simulink model "Prediction_3sAdvance_2output"  (R2016b)
settings: Solver=FixedStepAuto  StartTime=0.0  StopTime=length(lat_y)  FixedStep=1  RelTol=1e-3
StopFcn:
  | %%
  | scrsz = get(groot,'ScreenSize');
  | figure('Position',[40 scrsz(4)*0.1 scrsz(3)*0.8 scrsz(4)*0.8])
  | 
  | lng_margin = (max(LOCATIONLongitude(indices))-min(LOCATIONLongitude(indices)))*0.01;
  | lat_margin = (max(LOCATIONLatitude(indices))-min(LOCATIONLatitude(indices)))*0.01;
  | 
  | live_plot_title = ['Pedestrian Path Neural Network Prediction' newline ...
  |     'Green Rectangle:Current Position, Cyan Rectangle:Future Position' newline ...
  |     'blue line:predicted, green line:actual path'];
  | 
  | %occupy space on google map to plot the predicted trajectory
  | annotation('textbox', [0.7 0.9 0.1 0.1],'String', live_plot_title,'EdgeColor', 'k','HorizontalAlignment', 'center','FontWeight','bold');
  | 
  | %plot for acutal pedestrian path
  | subplot(1,2,1);
  | actual_lng = LOCATIONLongitude(indices);
  | actual_lat = LOCATIONLatitude(indices);
  | plot(actual_lng,actual_lat,'g','linewidth',2); hold on;
  | plot_google_map('MapType','satellite');
  | xlim([min(actual_lng)-lng_margin max(actual_lng)+lng_margin]);
  | ylim([min(actual_lat)-lat_margin max(actual_lat)+lat_margin]);
  | title('Actual Pedestrian Path');xlabel('Longitude');ylabel('Latitude');
  | 
  | 
  | predict_y = out_x.signals.values;
  | predict_x = out_y.signals.values;
  | 
  | %convert the predicted path to the latitude and longitude
  | [predict_lat,predict_lng] = utm2ll(predict_y + x_init, predict_x + y_init,zone);
  | subplot(1,2,2);
  | title('Predicted Pedestrian Path');xlabel('Longitude');ylabel('Latitude');
  | lat_lim = [min(predict_lat) min(predict_lat) max(predict_lat) max(predict_lat)];
  | long_lim = [max(predict_lng) min(predict_lng) min(predict_lng) max(predict_lng)];
  | scatter(long_lim, lat_lim);
  | plot_google_map('MapType','satellite');
  | xlim([min(predict_lng)-lng_margin max(predict_lng)+lng_margin]);
  | ylim([min(predict_lat)-lat_margin max(predict_lat)+lat_margin]);
  | for(i=1:1:length(actual_lat))
  |     plot(actual_lng(i),actual_lat(i),'gs','MarkerSize',10);hold on;
  |     plot(predict_lng(i),predict_lat(i),'bs','MarkerSize',10);hold on;
  | 
  |     RectPosCurr = [actual_lng(i)-lng_margin*2 actual_lat(i)-lat_margin*2 lng_margin*4 lat_margin*4];
  |     RectPosFuture = [predict_lng(i)-lng_margin*2 predict_lat(i)-lat_margin*2 lng_margin*4 lat_margin*4];
  |     showCurr = rectangle('Position',RectPosCurr,'FaceColor','g','Visible','on');
  |     showFuture = rectangle('Position',RectPosFuture,'FaceColor','c','Visible','on');
  |     pause(0.01/2);
  | 
  |     set(showCurr,'Visible','off');
  |     set(showFuture,'Visible','off');
  |     pause(0.01/2);
  | end
  | 
  | 
  | save('TestData_NNPred_3s.mat','indices','LOCATIONLatitude','LOCATIONLongitude','predict_lat','predict_lng');
values from neighbouring files (symbols this model uses):
  indices = [20 21 22 23 24 25 26 27 28 29 30 31 ... (1110 elements, 1110x1)]    [Circle.mat]    (also in DoubleEllipse.mat = [57 58 59 60 61 62 63 64 65 66 67 68 ... (2382 elements, 238; GPS_Path_Prediction.m = find(~isempty(orientation_temp)&~isnan(orientation_temp)); Rectangle.mat = [51 52 53 54 55 56 57 58 59 60 61 62 ... (1700 elements, 170; special_filter.m = find(variance<=var_threshold & abs(magnitude) <= mag_thresho)
  LOCATIONLatitude = [42.32249 42.32249 42.32249 42.32249 42.32249 42.32249 42.32249 42.32249 42.32249 42.32249 42.32249 42.32249 ... (1135 elements, 1135x1)]    [Circle.mat]    (also in DoubleEllipse.mat = [42.322384 42.322384 42.322384 42.322384 42.322384 42.322384; Rectangle.mat = [42.323025 42.323025 42.323025 42.323025 42.323025 42.323025)
  LOCATIONLongitude = [-83.479965 -83.479965 -83.479965 -83.479965 -83.479965 -83.479965 -83.479965 -83.479965 -83.479965 -83.479965 -83.479965 -83.479965 ... (1135 elements, 1135x1)]    [Circle.mat]    (also in DoubleEllipse.mat = [-83.47919 -83.47919 -83.47919 -83.47919 -83.47919 -83.47919; Rectangle.mat = [-83.47979 -83.47979 -83.47979 -83.47979 -83.47979 -83.47979)
libraries: neural x17
(part 2 of 2)

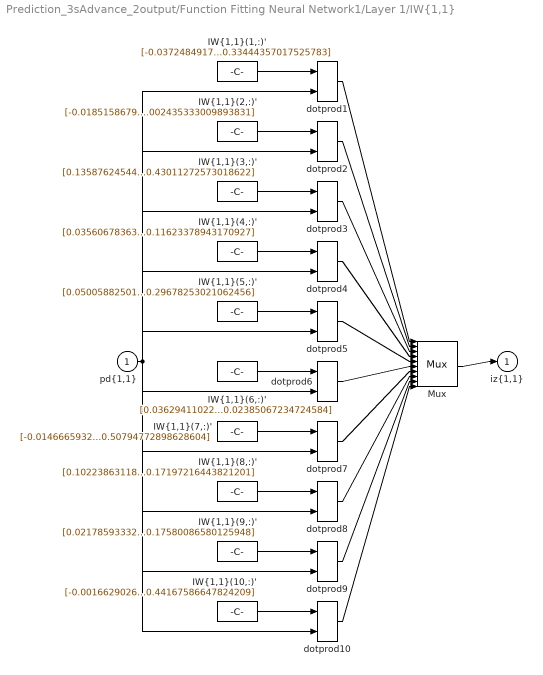
== system Prediction_3sAdvance_2output/Function Fitting Neural Network1/Layer 1/IW{1,1} ==
  "pd{1,1}" : Inport  PortDimensions=98
      mask Display: e = 0.06;c1 = [120 230 180]/255;c2 = ([120 230 180]+0)/(256+128);c3 = ([120 230 180]+128)/(256+128);patch([0 1 1 0],[0 0 1 1],c1);patch([0 1 1 1-e 1-e 0+e],[0 0 1 1-e 0+e 0+e],c2);patch([0 0 1 1-e 0+e 0+e],[0 1 1 1-e 1-e 0+e],c3);plot([0 1 1 0 0],[0 0 1 1 0]);
  "IW{1,1}(1,:)'" : Constant  Value=[-0.037248491787892045;0.0054460879972825669;-0.032907236588145455;0.0081200830673537269;0.045384948749954322;0.014503686240496656;0.03213178028993087;0.0044720544327022304;0.1328606211490925;-0.0022121594803582462;0.028994122142392876;-0.035971140027549996;0.012867042667458866;0.011984749837422535;-0.021689470658739135;-0.098691166617321593;0.013835297396100571;0.045570042540193985;0.006732817710215876;0.056374567113716509;0.043103145013547291;0.0094980051068001906;0.011375051456096234;0.044909003539689206;0.013443186350408389;0.064030515050383083;0.023608898902052266;-0.0018830103419206399;0.061923384001760527;0.099859366394465326;-0.035351467689058703;0.059571473168069197;0.050539807340897455;-0.0097345743458838955;-0.03019968727482451;-0.043083228725856432;-0.075672940267287103;-0.021341628750718045;-0.0075860255498702654;0.083882467573331537;0.087081548182975047;0.044326747243472769;0.04161843098207673;0.024419517359105761;0.067771261194288154;0.10793722049789942;0.098853911319223733;0.14510369382563093;0.14667611627198809;0.098747855953836922;0.055482620021514113;0.041358834886326398;-0.06234927403230036;0.02054383239817216;-0.0060832941492655933;-0.063800851461126837;0.025933913655796729;0.050253244099810558;0.17323753390638694;0.013583006031321749;0.047212997932893068;0.075090512042532781;0.020234443163722624;0.0096757232713807779;0.052770574120711317;0.070525108516196325;-0.038937279988646559;-0.041985340387868511;0.014003118123182268;-0.027139949440495883;0.035464437514537303;-0.020146467949284624;-0.029730945962615059;-0.033925780053117936;-0.062662865795619846;-0.073264534007386958;-0.092259914356993614;-0.12216892759248806;-0.036836270598460542;0.030334850772608789;-0.024565227656025427;-0.042277399900198631;-0.0024047230683458681;0.014120658740865528;-0.0072595459538706102;-0.061761095504444627;-0.06187148564013973;-0.10356580099254845;-0.067169875864027187;0.0070040934394714031;0.0071287719899211259;0.048236708391222453;0.037985710007260746;0.10302214241440466;0.11905881344586938;0.12569251526883041;0.16580876913423129;0.33444357017525783]
      mask Display: e = 0.06;c1 = [120 150 230]/255;c2 = ([120 150 230]+0)/383;c3 = ([120 150 230]+128)/383;patch([0 1 1 0],[0 0 1 1],c1);patch([0 1 1 1-e 1-e 0+e],[0 0 1 1-e 0+e 0+e],c2);patch([0 0 1 1-e 0+e 0+e],[0 1 1 1-e 1-e 0+e],c3);plot([0 1 1 0 0],[0 0 1 1 0]);disp('Weights');
  "IW{1,1}(10,:)'" : Constant  Value=[-0.0016629026063656727;-0.011225670780938314;0.01714849238849744;-0.014851048604781899;-0.020637093578709385;-0.0046831860505636659;0.043094815427376622;0.028144643783737999;-0.022275518567648131;-0.0054518287728863388;0.03074009069753697;0.025138591166365739;-0.0079854805933421528;-0.04352290978946536;0.0010432346396246478;0.074436831257383332;0.013522159226849562;-0.0341297472249463;0.023406280563916047;0.091245390177894556;0.03827735819353352;0.080714730073544433;0.040277637795607273;0.085186992106267831;0.0186755045141659;-0.0054963517695382066;0.0070899993972764665;0.02949082721780126;0.10821947711953832;0.10817926734261073;0.082409291320067232;0.031690910848052152;0.034667610327898127;0.0433582120696945;0.018192554323846189;0.056573488388800171;0.014924264980190824;0.020118047375342042;0.030480492656397247;-0.0058851918351701003;-0.076794887795094094;-0.055692543731693168;-0.0017313919310336671;-0.014917045039794821;0.012524053849874702;-0.078419463356555252;-0.059764956528005418;-0.028141054435656503;0.018383017379927775;0.025443583353570727;0.010694989338841221;0.0039818411387992731;0.042809605088047722;0.018337051314347801;-0.046626196567637515;0.0037444246905761658;-0.0020405572060482255;-0.043748333162415151;-0.060780149752281694;-0.0039068518534030299;0.05896696454326298;-0.02863175170986388;0.033266447694883572;0.041622866817240853;-0.08954756202660849;0.017972498221519192;0.03390177197352804;0.054709382453847911;0.05433729818294214;-0.0042915113923628718;-0.047063935588578409;-0.02706499899996518;-0.057794788791328849;-0.015379845884019749;0.022895306638709489;0.057993731050136714;0.078958851033474553;0.054172104572487355;0.038357924322599282;-0.083992107272182537;-0.072266815919457758;6.1798772163990078e-06;-0.07081353241630664;0.010229098049463453;0.018436384686728997;0.073894448949775676;0.029146559047782367;0.053097005701577576;0.02592954461261476;-0.1392726539051789;-0.078387592068944786;-0.09554649128959955;-0.12874955344751221;-0.10226641047758218;-0.15107489556282452;-0.16648423347524063;-0.2708673890968582;-0.44167586647824209]
      mask Display: e = 0.06;c1 = [120 150 230]/255;c2 = ([120 150 230]+0)/383;c3 = ([120 150 230]+128)/383;patch([0 1 1 0],[0 0 1 1],c1);patch([0 1 1 1-e 1-e 0+e],[0 0 1 1-e 0+e 0+e],c2);patch([0 0 1 1-e 0+e 0+e],[0 1 1 1-e 1-e 0+e],c3);plot([0 1 1 0 0],[0 0 1 1 0]);disp('Weights');
  "IW{1,1}(2,:)'" : Constant  Value=[-0.018515867974339798;0.0076899503655227701;0.01549069700479022;-0.0056572792377067574;-0.012941296175993957;0.0033684867282773841;-0.058734471901459022;-0.081499585394107829;-0.028289002835481376;-0.035714857870032694;0.025667867232901032;0.04701972373377955;-0.0042133746724056231;-0.040939734469384641;-0.081541047904027775;-0.035294479381303055;-0.025241872221598939;-0.044003899699484886;-0.061673568167941999;0.014271729195278368;0.039251376410087781;0.046993966092720267;-0.063891609263935056;-0.11313163856257076;-0.1658771793661056;-0.1489984542371538;-0.16679995745427703;-0.17934041911962106;-0.18280513882114119;-0.095936524801705836;-0.10069152341246847;-0.1258890389605237;-0.13539267595915977;-0.14402495236540552;-0.14208356430789368;-0.072830778023318485;-0.076229572602964174;-0.10200974763478331;-0.117850729273751;-0.024398371894119707;-0.061402312879435587;-0.05651051475020305;-0.00051209801424940873;0.0092792497807744866;0.031976932064244019;0.039163231932612605;0.10355035046087578;0.12284960076201655;0.21158867218529864;0.047482784905967378;0.065228424745243402;0.059897782952027571;0.080226172123634795;0.05566470801791959;0.090706225979411734;0.098944867731393382;0.068905625794264777;0.13976145424980396;0.21131314081599267;0.031745391815384078;-0.05505276308827943;0.014293117061868588;0.037198339502602117;0.062758768804144868;0.054681783297909493;0.051666561584193318;0.081668971795550535;0.11462921442882772;0.32986386475644031;0.036997138688802785;-0.013181832862036565;0.084037248324108471;0.057756839501518713;0.07889037953955623;0.0601386369901451;0.1018222445144861;0.13245023014536811;0.14926602137580236;0.24387994631514523;-0.058033518135738198;-0.045295437203196974;0.010683605378673021;-0.021991667219666146;0.0040487227994625485;-0.0072522018112378267;-0.0055938145531558405;0.04381260203260922;0.084441879469903974;0.25644765403914432;0.008448357593588399;0.024022196258855592;0.028951585693181837;0.042038473618834865;0.032302074150262969;0.026838544911972895;0.045227883905683615;0.073032635761526549;0.002435333009893831]
      mask Display: e = 0.06;c1 = [120 150 230]/255;c2 = ([120 150 230]+0)/383;c3 = ([120 150 230]+128)/383;patch([0 1 1 0],[0 0 1 1],c1);patch([0 1 1 1-e 1-e 0+e],[0 0 1 1-e 0+e 0+e],c2);patch([0 0 1 1-e 0+e 0+e],[0 1 1 1-e 1-e 0+e],c3);plot([0 1 1 0 0],[0 0 1 1 0]);disp('Weights');
  "IW{1,1}(3,:)'" : Constant  Value=[0.13587624544436069;0.049141070836930784;0.055226063647529307;-0.012024336315060894;0.029034721842293155;-0.0041841553803683021;-0.065110590519533496;-0.0050635145871141983;0.040305530529815912;-0.085086041805926646;-0.090753085285472365;-0.094194634308307393;-0.039192722872914643;-0.059810066311579785;0.015513472748620655;0.012009275529506782;-0.043981807150994111;-0.077587265971912206;-0.15548998679938819;-0.24987403328526672;-0.19804084126057198;-0.17565913085640739;-0.13977601925396552;-0.071775633359446422;-0.040272835600189856;-0.11407745658720843;-0.098303028907055404;-0.17288751490833559;-0.10522065490498507;-0.089892967049061634;-0.15403131387778668;-0.081779937720551907;-0.022034426415758288;0.01884725625518004;0.052770277999356845;0.03093008030701113;0.056756580220202753;0.06594354634264267;0.11632598695950128;0.068516598550003124;0.059536393304533461;0.092129347320588584;0.074913709596080291;0.054430210300128457;0.087264558634397277;0.079091055803260479;0.085051401799193779;0.037287353311588854;0.012666539134766626;-0.14012020554181653;-0.070051334847068603;-0.060773831053804538;0.013004994380231298;-0.014008098862541172;-0.037936218923967369;0.027244013025779147;-0.081009048385727381;-0.20417535790813271;-0.27273542717959298;-0.21118048832315597;-0.15657079304813487;-0.19154348051272566;-0.072217831691342022;-0.13419605969815465;-0.14409080429035978;-0.12215260942387618;-0.14080449342729862;-0.19174355199966939;-0.23874205581689281;-0.16896536250349556;-0.040501233782424088;0.04537096254121948;0.042332264815653019;0.063687965094504848;0.077026072108855481;0.053709327467266456;0.060106009911613419;-0.064670249270740748;-0.13381377122772231;-0.05098124119250879;-0.066430488971651713;-0.049535474912235977;0.00080231968539829109;-0.0090958125907286101;0.017502750704307284;0.0020256960728958001;0.013103620510808203;0.0018794618550559456;-0.1215060955417776;0.032972428012565801;0.020483431157685944;0.11723962277897426;0.11107314470112689;0.1874335444319373;0.23392080161571363;0.28071306377543098;0.36536466962570419;0.43011272573018622]
      mask Display: e = 0.06;c1 = [120 150 230]/255;c2 = ([120 150 230]+0)/383;c3 = ([120 150 230]+128)/383;patch([0 1 1 0],[0 0 1 1],c1);patch([0 1 1 1-e 1-e 0+e],[0 0 1 1-e 0+e 0+e],c2);patch([0 0 1 1-e 0+e 0+e],[0 1 1 1-e 1-e 0+e],c3);plot([0 1 1 0 0],[0 0 1 1 0]);disp('Weights');
  "IW{1,1}(4,:)'" : Constant  Value=[0.035606783631557504;-8.7920307566643552e-05;0.0077959643954650546;-0.026902507046974191;0.055430121324307691;-0.0081937769022633663;-0.019906801603008572;-0.017565781502400554;0.046813991938548988;-0.073208601225467254;-0.10161323200571563;-0.051330837516489369;-0.029012281240574062;-0.028052294075657895;-0.018270161675946285;-0.013769543175600253;0.022778808438588219;-0.0095418727838311856;-0.062534520451273667;-0.16162860103322177;-0.02839125452697229;0.038818876936792902;-0.0034962790707465663;0.044851793895644948;0.053178207180812023;0.061990968774601696;0.0050446935402055117;0.034178699305044177;0.10588014417961089;0.11956326788531846;0.20425031405267235;0.16405606467873152;0.14610633738655016;0.089798683528575618;0.087418745285612706;0.11500260140373852;0.079470205850699929;0.078160405812048944;0.027900751607239337;-0.025560766232941436;-0.094090816072839339;-0.042141551991293769;0.05901639672500518;0.040691879475591532;0.053787363822609929;0.042216007208548054;0.048387673558473156;0.06913261163375907;0.17816067291969345;0.1576713185227645;0.129922067015072;0.091200864970768583;0.060930988606987577;-0.010956761961097973;-0.055311056542727971;-0.011132434687715144;-0.06153535590517608;-0.13243463095951369;-0.19955970730551983;-0.22576929138787585;-0.23540660909952371;-0.14674720590313747;-0.12240047820282718;-0.10030002370112973;-0.10542871583418527;-0.14521324073126471;-0.17844998778519686;-0.36677533336408641;-0.33823936016763789;-0.29129894211593388;-0.289332280800773;-0.14220850820429379;-0.074582999652055337;-0.026680447939382124;-0.025778906285101599;0.004118716095315918;0.038496711872225468;-0.027659718751088871;0.0021762711750338737;-0.075576255254093186;-0.079810477521530282;-0.027772881627048111;0.012499026698608027;0.0082000081123978861;0.021694798721866596;-0.045196876928365388;-0.057483619182821417;-0.17512680000426883;-0.098411581131589446;-0.1837414194972174;-0.16401189957762166;-0.083125834629177095;-0.037564988463133393;-0.0064697206246631736;0.038046316375805488;0.053795825287118244;0.12973921102539035;0.11623378943170927]
      mask Display: e = 0.06;c1 = [120 150 230]/255;c2 = ([120 150 230]+0)/383;c3 = ([120 150 230]+128)/383;patch([0 1 1 0],[0 0 1 1],c1);patch([0 1 1 1-e 1-e 0+e],[0 0 1 1-e 0+e 0+e],c2);patch([0 0 1 1-e 0+e 0+e],[0 1 1 1-e 1-e 0+e],c3);plot([0 1 1 0 0],[0 0 1 1 0]);disp('Weights');
  "IW{1,1}(5,:)'" : Constant  Value=[0.050058825015330911;-0.0012653357721514285;0.034538905386114961;-0.0089377606265996241;0.00055185457157450263;0.028716340601122294;0.0079801906407940843;-0.045495655449408194;0.04903212752361312;-0.047442584364412857;0.01085405496138791;0.0039696743675070832;-0.10829696423943963;-0.11507296417008533;-0.1006916187242117;0.0072304873193762137;-0.0070198038464520359;-0.058760057489889314;0.065398623164374031;-0.035917083519191803;0.090562676150389973;0.10629228243770851;0.13429765641439287;0.10386240164693279;0.080837948128385781;0.022881057251614375;-0.021947611530623124;-0.021804302133922027;0.031072942275778778;-0.030446063342793282;-0.046646560789431871;-0.051629542562774168;-0.10581820304031463;-0.10980173691570538;-0.1308964798291026;-0.11654761923600809;-0.15267299201235127;-0.19546925099837423;-0.1140607288398868;-0.16559458645982331;-0.11283372853679467;-0.15367774445276097;-0.13635651783919578;-0.13753467451910104;-0.16584243315924277;-0.20303921452976351;-0.19214584685777183;-0.20321570190551377;-0.2776534551460817;-0.076180181496674992;-0.0025473866008764207;-0.071256638356988464;-0.014511365516534787;-0.026343766353206868;-0.055592068601036562;-0.039438910382926677;0.061541863800963992;0.048610001792157485;0.091072450948841421;0.015934665249430765;0.10721414601118008;0.12562602488722199;0.14617648697997296;0.14263743933781659;0.10361942488141937;0.16493857129751177;0.10064361611254671;0.10079502539515492;0.10869762397888007;0.0047085706518816767;-0.063207516262324653;-0.046679095438830011;-0.078800897801957731;-0.01925828839950719;-0.047901379372930791;-0.0096809452421214772;-0.033614754970806057;-0.002206098422528821;-0.042678487021817341;-0.11895473493421167;-0.13687664413830325;-0.10335031570448305;-0.092631636400148681;-0.050061928334915504;-0.11271154498971278;-0.053842161967614918;-0.12242795825287427;-0.11491296239191061;-0.22589475667958445;-0.19236680779187967;-0.25336304729864562;-0.24421160985511464;-0.23141079538680667;-0.22523512984473629;-0.21502591155537285;-0.32113772116854561;-0.31342712333284961;-0.29678253021062456]
      mask Display: e = 0.06;c1 = [120 150 230]/255;c2 = ([120 150 230]+0)/383;c3 = ([120 150 230]+128)/383;patch([0 1 1 0],[0 0 1 1],c1);patch([0 1 1 1-e 1-e 0+e],[0 0 1 1-e 0+e 0+e],c2);patch([0 0 1 1-e 0+e 0+e],[0 1 1 1-e 1-e 0+e],c3);plot([0 1 1 0 0],[0 0 1 1 0]);disp('Weights');
  "IW{1,1}(6,:)'" : Constant  Value=[0.036294110222280872;0.078796170074379418;0.048579716180394333;0.029244289310192888;0.027235092150712778;-0.030910566415148638;0.017589938715635575;0.077819079739231134;-0.0087185733058806197;0.0591595756626003;0.056277493880665538;0.068157807676395232;0.050072802450685336;0.0097377108828926393;-0.031357303137711512;0.040642525817573424;-0.019248081557384038;-0.0086311121682575327;-0.020976097996898403;-4.6612556843254944e-05;-0.016810053016620433;0.0011561770047757039;0.017340944138721202;-0.078866235730541398;-0.038973312525601302;-0.0021077233607033358;0.012216620132754341;0.11624884392460327;0.042525343289492465;0.00024963568421166633;0.097958686716235296;0.1044896119302359;0.074990858249646644;0.11753114014379942;0.14255312823070079;0.081536858660906902;0.11980864283949615;0.076464811217018272;0.11768083912366178;0.053040433000220877;0.071542565445890854;0.061184181214343838;0.068580045901338774;0.099053311571738051;0.067280443208284496;0.0071160854619471033;0.071633156194151087;0.050254524522790618;-0.1014827265327712;0.0077724080884053288;0.070219712452766245;0.045465455503656306;0.056391447889002279;-0.064793048136742276;0.0012113752311697468;-0.038150134401662879;-0.01917238666721521;0.035633616365967694;0.19173575257637138;0.10452066769211536;0.12306242916831635;0.0060892433529251564;-0.06482453628030875;-0.043758854212717552;0.059853881679656544;-0.020055661521191984;-0.11209882517192202;0.048397432977859686;-0.0014509675925307632;0.20499538105893558;0.11073499106249445;0.045751816712932734;-0.0073100694836159595;0.016905267946539196;0.12547688935575135;0.081686821840325552;0.085734675567429738;0.17620328903462648;0.1419606959089677;0.31580355105961361;0.29109174981011676;0.19899188574266435;0.21220310319535698;0.18750974150709493;0.15162092687987438;0.17150096652082733;0.086742438842789121;0.10228914434293929;-0.043299135787548855;0.24154249671365025;0.04904282370421801;0.009683197058250808;-0.034369901884648654;-0.12233370651460945;-0.032940987140248568;-0.14288660333844619;-0.10571383263686063;-0.02385067234724584]
      mask Display: e = 0.06;c1 = [120 150 230]/255;c2 = ([120 150 230]+0)/383;c3 = ([120 150 230]+128)/383;patch([0 1 1 0],[0 0 1 1],c1);patch([0 1 1 1-e 1-e 0+e],[0 0 1 1-e 0+e 0+e],c2);patch([0 0 1 1-e 0+e 0+e],[0 1 1 1-e 1-e 0+e],c3);plot([0 1 1 0 0],[0 0 1 1 0]);disp('Weights');
  "IW{1,1}(7,:)'" : Constant  Value=[-0.014666593294929673;-0.023849053736507236;0.10057629681203553;-0.033459367635151657;-0.017800969649502178;0.094328420690839951;-0.054952300257892134;-0.016408876540279452;-0.0010808271738179252;0.055856813019800361;0.028709089893787586;0.019198081511592736;0.0068891642880973365;-0.025526051979680491;-0.048521092247065044;-0.059371165239737934;-0.10626522110029785;-0.11173134731189713;-0.1567019531531002;-0.24381701032501404;-0.10620141751170588;-0.086642130807242909;-0.069984922800653188;-0.076803037864869944;-0.12880961747571362;-0.090158651735247841;-0.1121895976335499;-0.14436614507066087;-0.27362850791876014;-0.27224602476612014;-0.27653957217732689;-0.21609873164935664;-0.19591883771919844;-0.17982554515876314;-0.17779465142527737;-0.19930779523296477;-0.24919509672369416;-0.30167469463902602;-0.28400786220567803;-0.23036259657358774;-0.24391776145151073;-0.27528182346140972;-0.17723774254472699;-0.16956939145526093;-0.031673946971975203;0.011073978875322094;0.020780274924962053;0.078304658987660897;0.074408735737376733;0.020463221995305831;0.028546539783118052;0.023878048007705929;-0.052742891945343998;-0.0041387097469449781;-0.0080010659091822884;0.049683657186811045;-0.008826918879469365;0.08212713178374316;0.058714685912755096;0.011743116060139138;0.083325832271230776;0.033233503214297015;0.10589763416839633;0.097701861453665814;0.093614226190752936;0.14471650180075471;0.056109851744864263;0.071171805389080148;0.11662126683515273;0.084748222610678922;0.075889465048841906;0.022267953473523745;0.066044314721637493;0.070828092648408891;0.0067455649045431399;0.00823408814189471;-0.026556609470202729;-0.021764672041887471;0.035304696252847448;0.11604041970700579;0.04269389457981404;0.066776800334655245;0.11990162670126163;0.070806657605776188;0.013077728324594976;-0.011691177453661585;-0.01301891928728505;-0.16273344593329905;-0.12654502534015566;-0.19344433744542158;-0.18684895184911407;-0.26380517021195582;-0.30073548111838166;-0.3851543861164014;-0.39537862603135465;-0.38613876049065232;-0.48589585493548682;-0.50794772898628604]
      mask Display: e = 0.06;c1 = [120 150 230]/255;c2 = ([120 150 230]+0)/383;c3 = ([120 150 230]+128)/383;patch([0 1 1 0],[0 0 1 1],c1);patch([0 1 1 1-e 1-e 0+e],[0 0 1 1-e 0+e 0+e],c2);patch([0 0 1 1-e 0+e 0+e],[0 1 1 1-e 1-e 0+e],c3);plot([0 1 1 0 0],[0 0 1 1 0]);disp('Weights');
  "IW{1,1}(8,:)'" : Constant  Value=[0.10223863118349989;0.0098571802114627936;0.04812774276089566;-0.039278366808806746;0.0085449758935093531;-0.038266944221382028;-0.021816223534438649;0.0070492876737840403;-0.013828226632906754;0.071243257158375872;0.15687340687466017;0.026800003993120981;0.023074786424193777;0.0018172048651379454;-0.064247142922570152;0.0011984443015128478;-0.0016245895527836225;0.078675538136328022;0.05844144218268494;0.030221948655630989;0.037741836007381929;0.01511081508741486;0.033992878475336108;0.036624300291578829;0.036204100165814004;0.059789359542022427;0.13579025568880979;0.13547600669332444;0.062916187976159846;0.1467524817844639;0.047588295334307681;0.032779868744189783;0.030330742973224044;0.040649539213156706;0.073979198656162856;0.073117258907993685;0.044187137741152571;0.050759396469065882;0.11021176566343573;0.16170538973563484;0.11264862693875027;0.10156801866429757;0.13624643720797799;0.028059088759564164;0.043351606224381209;0.0081951031800280415;-0.032976723995227192;-0.0612812482562545;-0.09538225980030228;0.043982489143358429;-0.0002126735906692599;0.02356713661705219;0.0146041771394249;0.013403766838228423;0.015983309094350615;0.010728228551735391;-0.02015689082760546;0.077892366151023296;0.12898781441744472;0.15142186888409101;0.10009076456412259;0.055198497248916165;0.046313498315838822;0.046054446786903222;0.059713526932312723;-0.028853314323944369;0.065582389959090062;0.10983109368380314;0.09507448486312059;0.046173298735169989;-0.031191632758557946;-0.065131076427941748;-0.015622935372650387;-0.035522017545004898;0.020479103218939199;-0.0038704509394039814;0.054600165253808099;0.16433188779911326;0.1156722525253403;0.11444477445154674;0.085626237064705651;0.055026955722257645;0.0015026683588577037;-0.002796496658419708;0.0354929030502096;-0.039132148960143207;0.027131413852166133;0.12937587056249966;0.080881034026606902;0.01049817547726589;-0.038086295674814058;-0.015305335650777414;-0.020979655433616816;-0.11054190192980058;-0.083493088473367519;-0.071503080911199959;-0.12350987644581111;-0.17197216443821201]
      mask Display: e = 0.06;c1 = [120 150 230]/255;c2 = ([120 150 230]+0)/383;c3 = ([120 150 230]+128)/383;patch([0 1 1 0],[0 0 1 1],c1);patch([0 1 1 1-e 1-e 0+e],[0 0 1 1-e 0+e 0+e],c2);patch([0 0 1 1-e 0+e 0+e],[0 1 1 1-e 1-e 0+e],c3);plot([0 1 1 0 0],[0 0 1 1 0]);disp('Weights');
  "IW{1,1}(9,:)'" : Constant  Value=[0.021785933320828003;-0.0042439322084072209;0.062227612970194301;-0.040443602470480587;0.018076347409015953;-0.029587872594636019;-0.016013953321805725;-0.012620224272422749;0.086115385942117484;0.044885285366862995;-0.032821585277130513;-0.077671251694661061;-0.090606407822113877;-0.07559559920883159;-0.023791610703226239;-0.070558567673209227;-0.042854885421490657;-0.095855128000128229;-0.08211984202986726;0.0043518403431289723;-0.087790025045141426;-0.04038065808561684;-0.048061059436495544;-0.015302492285995312;-0.025828983194868899;0.016696160266914808;-0.0071027871197843432;-0.005552367534423573;0.11944558293146294;0.019388562906870473;0.015063132963555633;0.024926072000389692;0.0045193517097218633;0.04844520219302733;0.0043814647219027987;0.04514001131872044;0.052076949587895535;0.14490350930359391;0.18937331825487999;0.19312125088285115;0.17369744685204705;0.16813607865925409;0.14381321960028798;0.18520761590440435;0.1872422387306614;0.22390691212265709;0.25130128478851088;0.27374812824770001;0.42354617349692819;-0.016773152574865863;0.0052655593635517802;0.0065894628116083577;-0.029374045010493306;0.041977880563526561;-0.052913606343304373;-0.032723747129068836;-0.049574161064928103;-0.089548655385323708;0.01161043480248408;-0.0932952186572545;-0.0092363127152356207;-0.071142688454014835;0.026216999541976656;-0.035735567344781977;-0.096779543546836003;-0.0040969664106524578;-0.028625099899752881;-0.050264341014157242;-0.079878290075863195;-0.11859165015597516;-0.071522487258523143;-0.03354238110697589;-0.012810937097929097;0.034694868644078433;0.059965623592574728;0.053280753326303748;0.035473941295536673;0.054779716976357549;0.013201464289431055;-0.11068303163935853;-0.13340231250427817;-0.081931463035098767;-0.048985638247577186;-0.076269856697503607;-0.050987793884853257;-0.031213560347318831;-0.059841757339233137;-0.14779522726410463;-0.053225139452153195;-0.099287367327447876;-0.019394680534002871;-0.023067790472029684;0.062079140653176323;0.13064370661833319;0.13340893989808447;0.1584160890676338;0.15251437830300138;0.17580086580125948]
      mask Display: e = 0.06;c1 = [120 150 230]/255;c2 = ([120 150 230]+0)/383;c3 = ([120 150 230]+128)/383;patch([0 1 1 0],[0 0 1 1],c1);patch([0 1 1 1-e 1-e 0+e],[0 0 1 1-e 0+e 0+e],c2);patch([0 0 1 1-e 0+e 0+e],[0 1 1 1-e 1-e 0+e],c3);plot([0 1 1 0 0],[0 0 1 1 0]);disp('Weights');
  Mux : Mux  Inputs=10
      mask Display: e = 0.06;c1 = [120 150 230]/255;c2 = ([120 150 230]+0)/383;c3 = ([120 150 230]+128)/383;patch([0 1 1 0],[0 0 1 1],c1);patch([0 1 1 1-e 1-e 0+e],[0 0 1 1-e 0+e 0+e],c2);patch([0 0 1 1-e 0+e 0+e],[0 1 1 1-e 1-e 0+e],c3);plot([0 1 1 0 0],[0 0 1 1 0]);disp('Mux');
  dotprod{1..10} (10 alike) : neural/Weight Functions/dotprod
  "iz{1,1}" : Outport
      mask Display: e = 0.06;c1 = [120 230 180]/255;c2 = ([120 230 180]+0)/(256+128);c3 = ([120 230 180]+128)/(256+128);patch([0 1 1 0],[0 0 1 1],c1);patch([0 1 1 1-e 1-e 0+e],[0 0 1 1-e 0+e 0+e],c2);patch([0 0 1 1-e 0+e 0+e],[0 1 1 1-e 1-e 0+e],c3);plot([0 1 1 0 0],[0 0 1 1 0]);
  wires:
  "IW{1,1}(1,:)'"/1 -> dotprod1/1
  "pd{1,1}"/1 -> dotprod1/2, dotprod2/2, dotprod3/2, dotprod4/2, dotprod5/2, dotprod6/2, dotprod7/2, dotprod8/2, dotprod9/2, dotprod10/2
  dotprod1/1 -> Mux/1
  "IW{1,1}(2,:)'"/1 -> dotprod2/1
  dotprod2/1 -> Mux/2
  "IW{1,1}(3,:)'"/1 -> dotprod3/1
  dotprod3/1 -> Mux/3
  "IW{1,1}(4,:)'"/1 -> dotprod4/1
  dotprod4/1 -> Mux/4
  "IW{1,1}(5,:)'"/1 -> dotprod5/1
  dotprod5/1 -> Mux/5
  "IW{1,1}(6,:)'"/1 -> dotprod6/1
  dotprod6/1 -> Mux/6
  "IW{1,1}(7,:)'"/1 -> dotprod7/1
  dotprod7/1 -> Mux/7
  "IW{1,1}(8,:)'"/1 -> dotprod8/1
  dotprod8/1 -> Mux/8
  "IW{1,1}(9,:)'"/1 -> dotprod9/1
  dotprod9/1 -> Mux/9
  "IW{1,1}(10,:)'"/1 -> dotprod10/1
  dotprod10/1 -> Mux/10
  Mux/1 -> "iz{1,1}"/1

== system Prediction_3sAdvance_2output/Function Fitting Neural Network1/Layer 2/Delays 1 ==
  "p{2}" : Inport  PortDimensions=10
      mask Display: e = 0.06;c1 = [120 230 180]/255;c2 = ([120 230 180]+0)/(256+128);c3 = ([120 230 180]+128)/(256+128);patch([0 1 1 0],[0 0 1 1],c1);patch([0 1 1 1-e 1-e 0+e],[0 0 1 1-e 0+e 0+e],c2);patch([0 0 1 1-e 0+e 0+e],[0 1 1 1-e 1-e 0+e],c3);plot([0 1 1 0 0],[0 0 1 1 0]);
  mux : Mux  Inputs=1
      mask Display: e = 0.06;c1 = [120 150 230]/255;c2 = ([120 150 230]+0)/383;c3 = ([120 150 230]+128)/383;patch([0 1 1 0],[0 0 1 1],c1);patch([0 1 1 1-e 1-e 0+e],[0 0 1 1-e 0+e 0+e],c2);patch([0 0 1 1-e 0+e 0+e],[0 1 1 1-e 1-e 0+e],c3);plot([0 1 1 0 0],[0 0 1 1 0]);disp('Mux')
  "pd{2,1}" : Outport
      mask Display: e = 0.06;c1 = [120 230 180]/255;c2 = ([120 230 180]+0)/(256+128);c3 = ([120 230 180]+128)/(256+128);patch([0 1 1 0],[0 0 1 1],c1);patch([0 1 1 1-e 1-e 0+e],[0 0 1 1-e 0+e 0+e],c2);patch([0 0 1 1-e 0+e 0+e],[0 1 1 1-e 1-e 0+e],c3);plot([0 1 1 0 0],[0 0 1 1 0]);
  wires:
  "p{2}"/1 -> mux/1
  mux/1 -> "pd{2,1}"/1

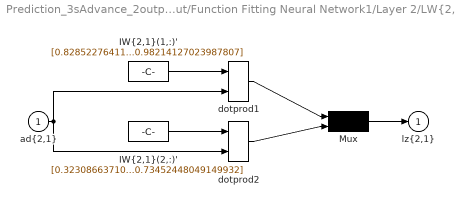
== system Prediction_3sAdvance_2output/Function Fitting Neural Network1/Layer 2/LW{2,1} ==
  "ad{2,1}" : Inport  PortDimensions=10
      mask Display: e = 0.06;c1 = [120 230 180]/255;c2 = ([120 230 180]+0)/(256+128);c3 = ([120 230 180]+128)/(256+128);patch([0 1 1 0],[0 0 1 1],c1);patch([0 1 1 1-e 1-e 0+e],[0 0 1 1-e 0+e 0+e],c2);patch([0 0 1 1-e 0+e 0+e],[0 1 1 1-e 1-e 0+e],c3);plot([0 1 1 0 0],[0 0 1 1 0]);
  "IW{2,1}(1,:)'" : Constant  Value=[0.82852276411321446;-0.088818652246628521;0.71793599586208234;-0.76745116459049201;-0.34136652448409299;-0.56793713989179806;0.44364880690398062;0.68019782282146046;-0.68520208370134339;0.98214127023987807]
      mask Display: e = 0.06;c1 = [120 150 230]/255;c2 = ([120 150 230]+0)/383;c3 = ([120 150 230]+128)/383;patch([0 1 1 0],[0 0 1 1],c1);patch([0 1 1 1-e 1-e 0+e],[0 0 1 1-e 0+e 0+e],c2);patch([0 0 1 1-e 0+e 0+e],[0 1 1 1-e 1-e 0+e],c3);plot([0 1 1 0 0],[0 0 1 1 0]);disp('weights');
  "IW{2,1}(2,:)'" : Constant  Value=[0.32308663710512991;0.47175687668311028;0.11914041449610929;0.26225639434209297;-0.6250403310859185;-0.76848980320195626;0.4039900232959206;0.3551121129197215;-0.17765714275594566;0.73452448049149932]
      mask Display: e = 0.06;c1 = [120 150 230]/255;c2 = ([120 150 230]+0)/383;c3 = ([120 150 230]+128)/383;patch([0 1 1 0],[0 0 1 1],c1);patch([0 1 1 1-e 1-e 0+e],[0 0 1 1-e 0+e 0+e],c2);patch([0 0 1 1-e 0+e 0+e],[0 1 1 1-e 1-e 0+e],c3);plot([0 1 1 0 0],[0 0 1 1 0]);disp('weights');
  Mux : Mux  Inputs=2
      mask Display: e = 0.06;c1 = [120 150 230]/255;c2 = ([120 150 230]+0)/383;c3 = ([120 150 230]+128)/383;patch([0 1 1 0],[0 0 1 1],c1);patch([0 1 1 1-e 1-e 0+e],[0 0 1 1-e 0+e 0+e],c2);patch([0 0 1 1-e 0+e 0+e],[0 1 1 1-e 1-e 0+e],c3);plot([0 1 1 0 0],[0 0 1 1 0]);disp('Mux');
  dotprod1 : neural/Weight Functions/dotprod
  dotprod2 : neural/Weight Functions/dotprod
  "lz{2,1}" : Outport
      mask Display: e = 0.06;c1 = [120 230 180]/255;c2 = ([120 230 180]+0)/(256+128);c3 = ([120 230 180]+128)/(256+128);patch([0 1 1 0],[0 0 1 1],c1);patch([0 1 1 1-e 1-e 0+e],[0 0 1 1-e 0+e 0+e],c2);patch([0 0 1 1-e 0+e 0+e],[0 1 1 1-e 1-e 0+e],c3);plot([0 1 1 0 0],[0 0 1 1 0]);
  wires:
  "IW{2,1}(1,:)'"/1 -> dotprod1/1
  "ad{2,1}"/1 -> dotprod1/2, dotprod2/2
  dotprod1/1 -> Mux/1
  "IW{2,1}(2,:)'"/1 -> dotprod2/1
  dotprod2/1 -> Mux/2
  Mux/1 -> "lz{2,1}"/1
